simulink model "KINARM_Dyn_Inv"  (Simulink 8.7)
settings: Solver=ode45  StartTime=tSimStart  StopTime=tSimEnd  FixedStep=0.005  RelTol=1e-24  AbsTol=1e-24  SampleTimeConstraint=STIndependent
undefined symbols (not defined in the file or in its folder): g, IeR, IsR, iStep, IwR, me, ms, mw, nIC
libraries: mblibv1 x28
Description:
  | MSB - Demo 2
settings Model: Creator=arnav  LastModifiedBy=LAB  ExtModeAutoUpdateStatusClock=off
settings SolverCC: InitialStep=iStep  ShapePreserveControl=EnableAll  ZeroCrossControl=EnableAll  ZeroCrossAlgorithm=Adaptive
settings DataIOCC: ExternalInput=[smpltime]  SignalLoggingSaveFormat=ModelDataLogs  SaveOutput=off  SignalLogging=off  DSMLogging=off  SaveTime=off  SignalLoggingName=sigsOut  Refine=5
settings OptimizationCC: BooleanDataType=off  ExpressionDepthLimit=2147483647  InitFltsAndDblsToZero=on
settings DebuggingCC: SaveWithParameterizedLinksMsg=none  CheckExecutionContextPreStartOutputMsg=on  CheckExecutionContextRuntimeOutputMsg=on  SignalResolutionControl=TryResolveAllWithWarning  MultiTaskDSMMsg=warning  MultiTaskCondExecSysMsg=none  FcnCallInpInsideContextMsg=UseLocalSettings  UnconnectedInputMsg=none  UnconnectedOutputMsg=none  UnconnectedLineMsg=none  StateNameClashWarn=warning
settings HardwareCC: TargetUnknown=on
settings GRTTargetCC: TargetFcnLib=ansi_tfl_tmw.mat  CombineOutputUpdateFcns=off  GRTInterface=on
settings ConfigurationSet: Description=SimMechanics 2G

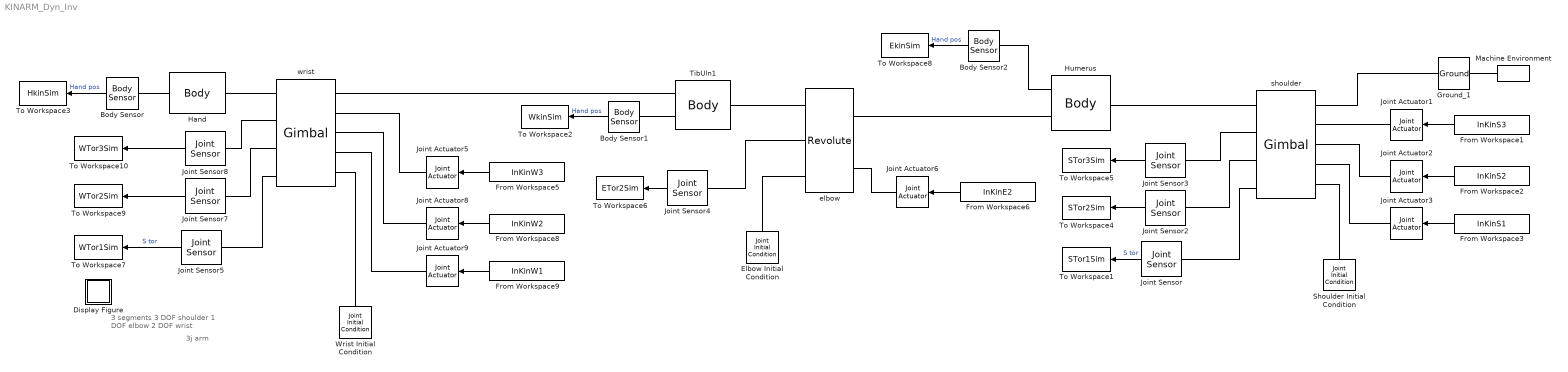
== system KINARM_Dyn_Inv ==
  note: 3j arm
  note: 3 segments
      | 3 DOF shoulder
      | 1 DOF elbow
      | 2 DOF wrist
  Body Sensor : mblibv1/Sensors &  Actuators/Body Sensor  UpdateFromCAD=off  PhysicalDomain=Mechanical  PortType=blob  Muxed=on  Pose=off  Angle=on  AngleUnits=deg  ArcVelocity=off  ArcVelocityUnits=deg/s  ArcAcceleration=off  ArcAccelerationUnits=deg/s^2  CoordPosition=on  CoordPositionUnits=m  Velocity=off  VelocityUnits=m/s  Acceleration=off  AccelerationUnits=m/s^2  Quaternion=on  QuaternionDT=off  QuaternionDDT=off  QuaternionUnits=off  OutputVector=[ 3 ]  ActiveIO=on  Width=3  DialogClass=MechanicalSensorBlock  ReferenceFrame=Absolute (World)
  Body Sensor1 : mblibv1/Sensors &  Actuators/Body Sensor  UpdateFromCAD=off  PhysicalDomain=Mechanical  PortType=blob  Muxed=on  Pose=off  Angle=on  AngleUnits=deg  ArcVelocity=off  ArcVelocityUnits=deg/s  ArcAcceleration=off  ArcAccelerationUnits=deg/s^2  CoordPosition=on  CoordPositionUnits=m  Velocity=off  VelocityUnits=m/s  Acceleration=off  AccelerationUnits=m/s^2  Quaternion=on  QuaternionDT=off  QuaternionDDT=off  QuaternionUnits=off  OutputVector=[ 3 ]  ActiveIO=on  Width=3  DialogClass=MechanicalSensorBlock  ReferenceFrame=Absolute (World)
  Body Sensor2 : mblibv1/Sensors &  Actuators/Body Sensor  UpdateFromCAD=off  PhysicalDomain=Mechanical  PortType=blob  Muxed=on  Pose=off  Angle=on  AngleUnits=deg  ArcVelocity=off  ArcVelocityUnits=deg/s  ArcAcceleration=off  ArcAccelerationUnits=deg/s^2  CoordPosition=on  CoordPositionUnits=m  Velocity=off  VelocityUnits=m/s  Acceleration=off  AccelerationUnits=m/s^2  Quaternion=on  QuaternionDT=off  QuaternionDDT=off  QuaternionUnits=off  OutputVector=[ 3 ]  ActiveIO=on  Width=3  DialogClass=MechanicalSensorBlock  ReferenceFrame=Absolute (World)
  Display Figure : Subsystem  Tag=Help  Description="Help callback for four bar model: mech_four_bar.  Opens Help browser to Type 19 marker at documentation for this tutorial model."  mask(Help callback){}
      settings: OpenFcn=pmhelpview([docroot '/toolbox/physmod/mech/mech.map'], 'mech_four_bar_help');
      mask Display: image(imread('info.bmp'))
  Elbow Initial Condition : mblibv1/Sensors &  Actuators/Joint Initial Condition  UpdateFromCAD=off  LeftPortType=blob  RightPortType=blob  PhysicalDomain=mechanical  DialogClass=InitialConditionBlock  InitialConditions=P1$false$0$m$deg$0$m/s$deg/s#P2$false$0$m$deg$0$m/s$deg/s#P3$false$0$m$deg$0$m/s$deg/s#R1$true$nIC(4,1)$m$rad$nIC(4,2)$m/s$rad/s#R2$false$nKin(1,1,5)$m$rad$nKin(1,2,5)$m/s$rad/s#R3$false$nKin(1,1,6)$m$rad$nKin(1,2,6)$m/s$rad/s#S$false$0$m$deg$0$m/s$deg/s  P1PIC=0  P1VIC=0  P2PIC=0  P2VIC=0  P3PIC=0  P3VIC=0  R1PIC=nIC(4,1)  R1VIC=nIC(4,2)  R2PIC=0  R2VIC=0  R3PIC=0  R3VIC=0  SPIC=0  SVIC=0
  From Workspace1 : FromWorkspace  VariableName=InKinS3  SampleTime=iStep  OutputAfterFinalValue=Holding final value
  From Workspace2 : FromWorkspace  VariableName=InKinS2  SampleTime=iStep  OutputAfterFinalValue=Holding final value
  From Workspace3 : FromWorkspace  VariableName=InKinS1  SampleTime=iStep  OutputAfterFinalValue=Holding final value
  From Workspace5 : FromWorkspace  VariableName=InKinW3  SampleTime=iStep  OutputAfterFinalValue=Holding final value
  From Workspace6 : FromWorkspace  VariableName=InKinE2  SampleTime=iStep  OutputAfterFinalValue=Holding final value
  From Workspace8 : FromWorkspace  VariableName=InKinW2  SampleTime=iStep  OutputAfterFinalValue=Holding final value
  From Workspace9 : FromWorkspace  VariableName=InKinW1  SampleTime=iStep  OutputAfterFinalValue=Holding final value
  Ground_1 : mblibv1/Bodies/Ground  UpdateFromCAD=off  LeftPortType=env  RightPortType=workingframe  PhysicalDomain=Mechanical  DialogClass=GroundBlock  CoordPosition=Spos  CoordPositionUnits=m  StateVectorMgrId=0  MachineId=[1 0]  ShowEnvPort=on  ParameterChecksum=[490472178, 4116704370, 4112686805, 3275683724]  TopologyChecksum=[4125622607, 929092055, 1872909337, 165519805]
  Hand : mblibv1/Bodies/Body  LConnTagsString=CS4  RConnTagsString=CS3  UpdateFromCAD=off  DialogClass=MechanicalBodyBlock  Mass=mw  MassUnits=kg  InertiaUnits=kg*m^2  Inertia=IwR  Shape=Cylinder  ShapeDims=[1 1]  ShapeUnits=m  ShapeUse=false  Density=1  DensityUnits=kg/m^3  DensityUse=false  GraphicsMode=MACHINE_DEFAULT  BodyColorSelMode=MACHINE_DEFAULT  BodyColor=[1 0 0]  AttachedToCS=CG  CG=Left$CG$HposCM$CS3$CS3$m$[0 0 0]$Euler X-Z-X$deg$WORLD$false$none  WorkingFrames=Right$CS3$Wpos$World$World$m$[0 0 0]$Euler X-Y-Z$deg$Adjoining$true$none#Left$CS4$Hpos$World$World$m$[0 0 0]$Euler X-Y-Z$deg$WORLD$true$none#Left$CS8$[0 0 0]$CS4$CS4$m$[0 0 0]$Euler X-Y-Z$deg$WORLD$false$none#Left$CS7$[0 0 0]$CS4$CS4$m$[0 0 0]$Euler X-Y-Z$deg$WORLD$false$none#Left$CS6$[0 0 0]$CS4$CS4$m$[0 0 0]$Euler X-Y-Z$deg$WORLD$false$none  CGPos=HposCM  CGRot=[0 0 0]  CS0Pos=[]  CS0Rot=[]  CS1Pos=[]  CS1Rot=[]  CS2Pos=[]  CS2Rot=[]  CS3Pos=Wpos  CS3Rot=[0 0 0]  CS4Pos=Hpos  CS4Rot=[0 0 0]  CS5Pos=[]  CS5Rot=[]  CS6Pos=[0 0 0]  CS6Rot=[0 0 0]  CS7Pos=[0 0 0]  CS7Rot=[0 0 0]  CS8Pos=[0 0 0]  CS8Rot=[0 0 0]  CS9Pos=[]  CS9Rot=[]  CS10Pos=[]  CS10Rot=[]  CS11Pos=[]  CS11Rot=[]  CS12Pos=[]  CS12Rot=[]  CS13Pos=[]  CS13Rot=[]  CS14Pos=[]  CS14Rot=[]  CS15Pos=[]  CS15Rot=[]  CS16Pos=[]  CS16Rot=[]  CS17Pos=[]  CS17Rot=[]  CS18Pos=[]  CS18Rot=[]  CS19Pos=[]  CS19Rot=[]  CS20Pos=[]  CS20Rot=[]
  Humerus : mblibv1/Bodies/Body  LConnTagsString=CS1  RConnTagsString=CS3|CS2  UpdateFromCAD=off  DialogClass=MechanicalBodyBlock  Mass=ms  MassUnits=kg  InertiaUnits=kg*m^2  Inertia=IsR  Shape=Cylinder  ShapeDims=[1 1]  ShapeUnits=m  ShapeUse=false  Density=1  DensityUnits=kg/m^3  DensityUse=false  GraphicsMode=MACHINE_DEFAULT  BodyColorSelMode=MACHINE_DEFAULT  BodyColor=[1 0 0]  AttachedToCS=CG  CG=Left$CG$EposCM$World$World$m$[0 0 0]$Euler X-Y-Z$deg$WORLD$false$none  WorkingFrames=Left$CS1$Spos$WORLD$WORLD$m$[0 0 0]$Euler X-Y-Z$deg$WORLD$true$none#Left$CS4$Spos$WORLD$WORLD$m$[0 0 0]$Euler X-Y-Z$deg$WORLD$false$none#Right$CS3$Epos$WORLD$WORLD$m$[0 0 0]$Euler X-Y-Z$deg$WORLD$true$none#Right$CS2$Epos$World$World$m$[0 0 0]$Euler X-Y-Z$deg$WORLD$true$none  CGPos=EposCM  CGRot=[0 0 0]  CS0Pos=[]  CS0Rot=[]  CS1Pos=Spos  CS1Rot=[0 0 0]  CS2Pos=Epos  CS2Rot=[0 0 0]  CS3Pos=Epos  CS3Rot=[0 0 0]  CS4Pos=Spos  CS4Rot=[0 0 0]  CS5Pos=[]  CS5Rot=[]  CS6Pos=[]  CS6Rot=[]  CS7Pos=[]  CS7Rot=[]  CS8Pos=[]  CS8Rot=[]  CS9Pos=[]  CS9Rot=[]  CS10Pos=[]  CS10Rot=[]  CS11Pos=[]  CS11Rot=[]  CS12Pos=[]  CS12Rot=[]  CS13Pos=[]  CS13Rot=[]  CS14Pos=[]  CS14Rot=[]  CS15Pos=[]  CS15Rot=[]  CS16Pos=[]  CS16Rot=[]  CS17Pos=[]  CS17Rot=[]  CS18Pos=[]  CS18Rot=[]  CS19Pos=[]  CS19Rot=[]  CS20Pos=[]  CS20Rot=[]
  Joint Actuator1 : mblibv1/Sensors &  Actuators/Joint Actuator  UpdateFromCAD=off  PhysicalDomain=Mechanical  PortType=blob  ActuationStyle=Motion  AngleUnits=rad  ArcVelocityUnits=rad/s  ArcAccelerationUnits=rad/s^2  CoordPositionUnits=m  VelocityUnits=m/s  AccelerationUnits=m/s^2  ForceUnits=N  TorqueUnits=N*m  ActiveIO=on  Width=3  DialogClass=MechanicalActuatorBlock  Primitive=R3  ReferenceFrame=Absolute (INERTIAL)
  Joint Actuator2 : mblibv1/Sensors &  Actuators/Joint Actuator  UpdateFromCAD=off  PhysicalDomain=Mechanical  PortType=blob  ActuationStyle=Motion  AngleUnits=rad  ArcVelocityUnits=rad/s  ArcAccelerationUnits=rad/s^2  CoordPositionUnits=m  VelocityUnits=m/s  AccelerationUnits=m/s^2  ForceUnits=N  TorqueUnits=N*m  ActiveIO=on  Width=3  DialogClass=MechanicalActuatorBlock  Primitive=R2  ReferenceFrame=Absolute (INERTIAL)
  Joint Actuator3 : mblibv1/Sensors &  Actuators/Joint Actuator  UpdateFromCAD=off  PhysicalDomain=Mechanical  PortType=blob  ActuationStyle=Motion  AngleUnits=rad  ArcVelocityUnits=rad/s  ArcAccelerationUnits=rad/s^2  CoordPositionUnits=m  VelocityUnits=m/s  AccelerationUnits=m/s^2  ForceUnits=N  TorqueUnits=N*m  ActiveIO=on  Width=3  DialogClass=MechanicalActuatorBlock  Primitive=R1  ReferenceFrame=Absolute (INERTIAL)
  Joint Actuator5 : mblibv1/Sensors &  Actuators/Joint Actuator  UpdateFromCAD=off  PhysicalDomain=Mechanical  PortType=blob  ActuationStyle=Motion  AngleUnits=rad  ArcVelocityUnits=rad/s  ArcAccelerationUnits=rad/s^2  CoordPositionUnits=m  VelocityUnits=m/s  AccelerationUnits=m/s^2  ForceUnits=N  TorqueUnits=N*m  ActiveIO=on  Width=3  DialogClass=MechanicalActuatorBlock  Primitive=R3  ReferenceFrame=Absolute (INERTIAL)
  Joint Actuator6 : mblibv1/Sensors &  Actuators/Joint Actuator  UpdateFromCAD=off  PhysicalDomain=Mechanical  PortType=blob  ActuationStyle=Motion  AngleUnits=rad  ArcVelocityUnits=rad/s  ArcAccelerationUnits=rad/s^2  CoordPositionUnits=m  VelocityUnits=m/s  AccelerationUnits=m/s^2  ForceUnits=N  TorqueUnits=N*m  ActiveIO=on  Width=3  DialogClass=MechanicalActuatorBlock  Primitive=R1  ReferenceFrame=Absolute (INERTIAL)
  Joint Actuator8 : mblibv1/Sensors &  Actuators/Joint Actuator  UpdateFromCAD=off  PhysicalDomain=Mechanical  PortType=blob  ActuationStyle=Motion  AngleUnits=rad  ArcVelocityUnits=rad/s  ArcAccelerationUnits=rad/s^2  CoordPositionUnits=m  VelocityUnits=m/s  AccelerationUnits=m/s^2  ForceUnits=N  TorqueUnits=N*m  ActiveIO=on  Width=3  DialogClass=MechanicalActuatorBlock  Primitive=R2  ReferenceFrame=Absolute (INERTIAL)
  Joint Actuator9 : mblibv1/Sensors &  Actuators/Joint Actuator  UpdateFromCAD=off  PhysicalDomain=Mechanical  PortType=blob  ActuationStyle=Motion  AngleUnits=rad  ArcVelocityUnits=rad/s  ArcAccelerationUnits=rad/s^2  CoordPositionUnits=m  VelocityUnits=m/s  AccelerationUnits=m/s^2  ForceUnits=N  TorqueUnits=N*m  ActiveIO=on  Width=3  DialogClass=MechanicalActuatorBlock  Primitive=R1  ReferenceFrame=Absolute (INERTIAL)
  Joint Sensor : mblibv1/Sensors &  Actuators/Joint Sensor  UpdateFromCAD=off  PhysicalDomain=Mechanical  PortType=blob  Muxed=off  Pose=off  Angle=off  AngleUnits=rad  ArcVelocity=off  ArcVelocityUnits=rad/s  ArcAcceleration=off  ArcAccelerationUnits=rad/s^2  CoordPosition=on  CoordPositionUnits=m  Velocity=off  VelocityUnits=m/s  Acceleration=off  AccelerationUnits=m/s^2  Quaternion=on  QuaternionDT=off  QuaternionDDT=off  QuaternionUnits=off  OutputVector=[ 1 1 ]  ActiveIO=on  Width=1  DialogClass=MechanicalSensorBlock  Primitive=R1  Force=off  ForceUnits=N  Torque=on  TorqueUnits=N*m  ReferenceFrame=Absolute (INERTIAL)  ReactionSensedSide=Base  ReactionReferenceFrame=Local (Body CS)  ReactionForce=off  ReactionForceUnits=N  ReactionMoment=off  ReactionMomentUnits=N*m
  Joint Sensor2 : mblibv1/Sensors &  Actuators/Joint Sensor  UpdateFromCAD=off  PhysicalDomain=Mechanical  PortType=blob  Muxed=off  Pose=off  Angle=off  AngleUnits=rad  ArcVelocity=off  ArcVelocityUnits=rad/s  ArcAcceleration=off  ArcAccelerationUnits=rad/s^2  CoordPosition=on  CoordPositionUnits=m  Velocity=off  VelocityUnits=m/s  Acceleration=off  AccelerationUnits=m/s^2  Quaternion=on  QuaternionDT=off  QuaternionDDT=off  QuaternionUnits=off  OutputVector=[ 1 1 ]  ActiveIO=on  Width=1  DialogClass=MechanicalSensorBlock  Primitive=R2  Force=off  ForceUnits=N  Torque=on  TorqueUnits=N*m  ReferenceFrame=Absolute (INERTIAL)  ReactionSensedSide=Base  ReactionReferenceFrame=Local (Body CS)  ReactionForce=off  ReactionForceUnits=N  ReactionMoment=off  ReactionMomentUnits=N*m
  Joint Sensor3 : mblibv1/Sensors &  Actuators/Joint Sensor  UpdateFromCAD=off  PhysicalDomain=Mechanical  PortType=blob  Muxed=off  Pose=off  Angle=off  AngleUnits=rad  ArcVelocity=off  ArcVelocityUnits=rad/s  ArcAcceleration=off  ArcAccelerationUnits=rad/s^2  CoordPosition=on  CoordPositionUnits=m  Velocity=off  VelocityUnits=m/s  Acceleration=off  AccelerationUnits=m/s^2  Quaternion=on  QuaternionDT=off  QuaternionDDT=off  QuaternionUnits=off  OutputVector=[ 1 1 ]  ActiveIO=on  Width=1  DialogClass=MechanicalSensorBlock  Primitive=R3  Force=off  ForceUnits=N  Torque=on  TorqueUnits=N*m  ReferenceFrame=Absolute (INERTIAL)  ReactionSensedSide=Base  ReactionReferenceFrame=Local (Body CS)  ReactionForce=off  ReactionForceUnits=N  ReactionMoment=off  ReactionMomentUnits=N*m
  Joint Sensor4 : mblibv1/Sensors &  Actuators/Joint Sensor  UpdateFromCAD=off  PhysicalDomain=Mechanical  PortType=blob  Muxed=off  Pose=off  Angle=off  AngleUnits=rad  ArcVelocity=off  ArcVelocityUnits=rad/s  ArcAcceleration=off  ArcAccelerationUnits=rad/s^2  CoordPosition=on  CoordPositionUnits=m  Velocity=off  VelocityUnits=m/s  Acceleration=off  AccelerationUnits=m/s^2  Quaternion=on  QuaternionDT=off  QuaternionDDT=off  QuaternionUnits=off  OutputVector=[ 1 1 ]  ActiveIO=on  Width=1  DialogClass=MechanicalSensorBlock  Primitive=R1  Force=off  ForceUnits=N  Torque=on  TorqueUnits=N*m  ReferenceFrame=Absolute (INERTIAL)  ReactionSensedSide=Base  ReactionReferenceFrame=Local (Body CS)  ReactionForce=off  ReactionForceUnits=N  ReactionMoment=off  ReactionMomentUnits=N*m
  Joint Sensor5 : mblibv1/Sensors &  Actuators/Joint Sensor  UpdateFromCAD=off  PhysicalDomain=Mechanical  PortType=blob  Muxed=off  Pose=off  Angle=off  AngleUnits=rad  ArcVelocity=off  ArcVelocityUnits=rad/s  ArcAcceleration=off  ArcAccelerationUnits=rad/s^2  CoordPosition=on  CoordPositionUnits=m  Velocity=off  VelocityUnits=m/s  Acceleration=off  AccelerationUnits=m/s^2  Quaternion=on  QuaternionDT=off  QuaternionDDT=off  QuaternionUnits=off  OutputVector=[ 1 1 ]  ActiveIO=on  Width=1  DialogClass=MechanicalSensorBlock  Primitive=R1  Force=off  ForceUnits=N  Torque=on  TorqueUnits=N*m  ReferenceFrame=Absolute (INERTIAL)  ReactionSensedSide=Base  ReactionReferenceFrame=Local (Body CS)  ReactionForce=off  ReactionForceUnits=N  ReactionMoment=off  ReactionMomentUnits=N*m
  Joint Sensor7 : mblibv1/Sensors &  Actuators/Joint Sensor  UpdateFromCAD=off  PhysicalDomain=Mechanical  PortType=blob  Muxed=off  Pose=off  Angle=off  AngleUnits=rad  ArcVelocity=off  ArcVelocityUnits=rad/s  ArcAcceleration=off  ArcAccelerationUnits=rad/s^2  CoordPosition=on  CoordPositionUnits=m  Velocity=off  VelocityUnits=m/s  Acceleration=off  AccelerationUnits=m/s^2  Quaternion=on  QuaternionDT=off  QuaternionDDT=off  QuaternionUnits=off  OutputVector=[ 1 1 ]  ActiveIO=on  Width=1  DialogClass=MechanicalSensorBlock  Primitive=R2  Force=off  ForceUnits=N  Torque=on  TorqueUnits=N*m  ReferenceFrame=Absolute (INERTIAL)  ReactionSensedSide=Base  ReactionReferenceFrame=Local (Body CS)  ReactionForce=off  ReactionForceUnits=N  ReactionMoment=off  ReactionMomentUnits=N*m
  Joint Sensor8 : mblibv1/Sensors &  Actuators/Joint Sensor  UpdateFromCAD=off  PhysicalDomain=Mechanical  PortType=blob  Muxed=off  Pose=off  Angle=off  AngleUnits=rad  ArcVelocity=off  ArcVelocityUnits=rad/s  ArcAcceleration=off  ArcAccelerationUnits=rad/s^2  CoordPosition=on  CoordPositionUnits=m  Velocity=off  VelocityUnits=m/s  Acceleration=off  AccelerationUnits=m/s^2  Quaternion=on  QuaternionDT=off  QuaternionDDT=off  QuaternionUnits=off  OutputVector=[ 1 1 ]  ActiveIO=on  Width=1  DialogClass=MechanicalSensorBlock  Primitive=R3  Force=off  ForceUnits=N  Torque=on  TorqueUnits=N*m  ReferenceFrame=Absolute (INERTIAL)  ReactionSensedSide=Base  ReactionReferenceFrame=Local (Body CS)  ReactionForce=off  ReactionForceUnits=N  ReactionMoment=off  ReactionMomentUnits=N*m
  Machine Environment : mblibv1/Bodies/Machine Environment  Tag=Factory ground  PortType=env  PhysicalDomain=Mechanical  DialogTemplateClass=MECH.MachineEnvironment  SyncWhenCopied=off  Gravity=[0 0 -g]  GravityUnits=m/s^2  GravityAsSignal=off  Dimensionality=3D Only  AnalysisType=Inverse dynamics  LinearAssemblyTolerance=1e-12  LinearAssemblyToleranceUnits=m  AngularAssemblyTolerance=1e-12  AngularAssemblyToleranceUnits=rad  ConstraintSolverType=Stabilizing  ConstraintRelTolerance=1e-4  ConstraintAbsTolerance=1e-4  UseRobustSingularityHandling=off  RedundancyAnalysisToleranceType=Automatically select tolerance  RedundancyAnalysisTolerance=1e-14  StatePerturbationType=Adaptive  PerturbationSize=1e-3  VisualizeMachine=off  BodyVisualizationType=Convex hull from body CS locations  BodyColorSelMode=Use model default  DefaultBodyColor=[1 0 0]
  Shoulder Initial Condition : mblibv1/Sensors &  Actuators/Joint Initial Condition  UpdateFromCAD=off  LeftPortType=blob  RightPortType=blob  PhysicalDomain=mechanical  DialogClass=InitialConditionBlock  InitialConditions=P1$false$0$m$deg$0$m/s$deg/s#P2$false$0$m$deg$0$m/s$deg/s#P3$false$0$m$deg$0$m/s$deg/s#R1$true$nIC(1,1)$m$rad$nIC(1,2)$m/s$rad/s#R2$true$nIC(2,1)$m$rad$nIC(2,2)$m/s$rad/s#R3$true$nIC(3,1)$m$rad$nIC(3,2)$m/s$rad/s#S$false$0$m$deg$0$m/s$deg/s  P1PIC=0  P1VIC=0  P2PIC=0  P2VIC=0  P3PIC=0  P3VIC=0  R1PIC=nIC(1,1)  R1VIC=nIC(1,2)  R2PIC=nIC(2,1)  R2VIC=nIC(2,2)  R3PIC=nIC(3,1)  R3VIC=nIC(3,2)  SPIC=0  SVIC=0
  TibUln1 : mblibv1/Bodies/Body  LConnTagsString=CS3  RConnTagsString=CS4|CS5  UpdateFromCAD=off  DialogClass=MechanicalBodyBlock  Mass=me  MassUnits=kg  InertiaUnits=kg*m^2  Inertia=IeR  Shape=Cylinder  ShapeDims=[1 1]  ShapeUnits=m  ShapeUse=false  Density=1  DensityUnits=kg/m^3  DensityUse=false  GraphicsMode=MACHINE_DEFAULT  BodyColorSelMode=MACHINE_DEFAULT  BodyColor=[1 0 0]  AttachedToCS=CG  CG=Left$CG$WposCM$CS3$CS3$m$[0 0 0]$Euler X-Z-X$deg$WORLD$false$none  WorkingFrames=Left$CS3$Epos$World$World$m$[0 0 0]$Euler X-Y-Z$deg$Adjoining$true$none#Right$CS4$Wpos$World$World$m$[0 0 0]$Euler X-Y-Z$deg$WORLD$true$none#Right$CS5$Wpos$World$World$m$[0 0 0]$Euler X-Y-Z$deg$WORLD$true$none  CGPos=WposCM  CGRot=[0 0 0]  CS0Pos=[]  CS0Rot=[]  CS1Pos=[]  CS1Rot=[]  CS2Pos=[]  CS2Rot=[]  CS3Pos=Epos  CS3Rot=[0 0 0]  CS4Pos=Wpos  CS4Rot=[0 0 0]  CS5Pos=Wpos  CS5Rot=[0 0 0]  CS6Pos=[]  CS6Rot=[]  CS7Pos=[]  CS7Rot=[]  CS8Pos=[]  CS8Rot=[]  CS9Pos=[]  CS9Rot=[]  CS10Pos=[]  CS10Rot=[]  CS11Pos=[]  CS11Rot=[]  CS12Pos=[]  CS12Rot=[]  CS13Pos=[]  CS13Rot=[]  CS14Pos=[]  CS14Rot=[]  CS15Pos=[]  CS15Rot=[]  CS16Pos=[]  CS16Rot=[]  CS17Pos=[]  CS17Rot=[]  CS18Pos=[]  CS18Rot=[]  CS19Pos=[]  CS19Rot=[]  CS20Pos=[]  CS20Rot=[]
  To Workspace1 : ToWorkspace  VariableName=STor1Sim  SaveFormat=Structure With Time  SampleTime=-1
      settings: Decimation=5
  To Workspace10 : ToWorkspace  VariableName=WTor3Sim  SaveFormat=Structure With Time  SampleTime=-1
      settings: Decimation=5
  To Workspace2 : ToWorkspace  VariableName=WkinSim  SampleTime=-1
      settings: Decimation=5
  To Workspace3 : ToWorkspace  VariableName=HkinSim  SampleTime=-1
      settings: Decimation=5
  To Workspace4 : ToWorkspace  VariableName=STor2Sim  SaveFormat=Structure With Time  SampleTime=-1
      settings: Decimation=5
  To Workspace5 : ToWorkspace  VariableName=STor3Sim  SaveFormat=Structure With Time  SampleTime=-1
      settings: Decimation=5
  To Workspace6 : ToWorkspace  VariableName=ETor2Sim  SaveFormat=Structure With Time  SampleTime=-1
      settings: Decimation=5
  To Workspace7 : ToWorkspace  VariableName=WTor1Sim  SaveFormat=Structure With Time  SampleTime=-1
      settings: Decimation=5
  To Workspace8 : ToWorkspace  VariableName=EkinSim  SampleTime=-1
      settings: Decimation=5
  To Workspace9 : ToWorkspace  VariableName=WTor2Sim  SaveFormat=Structure With Time  SampleTime=-1
      settings: Decimation=5
  Wrist Initial Condition : mblibv1/Sensors &  Actuators/Joint Initial Condition  UpdateFromCAD=off  LeftPortType=blob  RightPortType=blob  PhysicalDomain=mechanical  DialogClass=InitialConditionBlock  InitialConditions=P1$false$0$m$deg$0$m/s$deg/s#P2$false$0$m$deg$0$m/s$deg/s#P3$false$0$m$deg$0$m/s$deg/s#R1$true$nIC(5,1)$m$rad$nIC(5,2)$m/s$rad/s#R2$true$nIC(6,1)$m$rad$nIC(6,2)$m/s$rad/s#R3$true$nIC(7,1)$m$rad$nIC(7,2)$m/s$rad/s#S$false$0$m$deg$0$m/s$deg/s  P1PIC=0  P1VIC=0  P2PIC=0  P2VIC=0  P3PIC=0  P3VIC=0  R1PIC=nIC(5,1)  R1VIC=nIC(5,2)  R2PIC=nIC(6,1)  R2VIC=nIC(6,2)  R3PIC=nIC(7,1)  R3VIC=nIC(7,2)  SPIC=0  SVIC=0
  elbow : mblibv1/Joints/Revolute  LConnTagsString=__newl0|SA1|SA2  RConnTagsString=__newr0|SA1  UpdateFromCAD=off  NumSAPorts=3  CutJoint=off  MarkAsCut=off  Primitives=prismatic  PrimitiveProps=R1$Base$[1 0 0]$revolute  DialogClass=JointBlock  R1Axis=[1 0 0]
  shoulder : mblibv1/Joints/Gimbal  LConnTagsString=__newl0|SA1|SA2|SA3|SA4  RConnTagsString=__newr0|SA1|SA2|SA3  UpdateFromCAD=off  NumSAPorts=7  CutJoint=off  MarkAsCut=off  Primitives=prismatic_prismatic  PrimitiveProps=R1$Base$[1 0 0]$revolute#R2$Base$[0 1 0]$revolute#R3$Base$[0 0 1]$revolute  DialogClass=JointBlock  R1Axis=[1 0 0]  R2Axis=[0 1 0]  R3Axis=[0 0 1]
  wrist : mblibv1/Joints/Gimbal  LConnTagsString=__newl0|SA1|SA2|SA3|SA4  RConnTagsString=__newr0|SA1|SA2|SA3  UpdateFromCAD=off  NumSAPorts=7  CutJoint=off  MarkAsCut=off  Primitives=prismatic_prismatic  PrimitiveProps=R1$Base$[1 0 0]$revolute#R2$Base$[0 1 0]$revolute#R3$Base$[0 0 1]$revolute  DialogClass=JointBlock  R1Axis=[1 0 0]  R2Axis=[0 1 0]  R3Axis=[0 0 1]
  wires:
  Body Sensor/1 -> To Workspace3/1  "Hand pos"
  From Workspace1/1 -> Joint Actuator1/1
  Joint Sensor/1 -> To Workspace1/1  "S tor"
  From Workspace2/1 -> Joint Actuator2/1
  Joint Sensor2/1 -> To Workspace4/1
  From Workspace3/1 -> Joint Actuator3/1
  Joint Sensor3/1 -> To Workspace5/1
  From Workspace6/1 -> Joint Actuator6/1
  Joint Sensor4/1 -> To Workspace6/1
  From Workspace5/1 -> Joint Actuator5/1
  Joint Sensor5/1 -> To Workspace7/1  "S tor"
  From Workspace8/1 -> Joint Actuator8/1
  Joint Sensor7/1 -> To Workspace9/1
  From Workspace9/1 -> Joint Actuator9/1
  Joint Sensor8/1 -> To Workspace10/1
  Body Sensor1/1 -> To Workspace2/1  "Hand pos"
  Body Sensor2/1 -> To Workspace8/1  "Hand pos"
  connections:
  Machine Environment/RConn1 -- Ground_1/LConn1
  Ground_1/RConn1 -- shoulder/LConn1
  Joint Sensor/LConn1 -- shoulder/RConn4
  Joint Sensor2/LConn1 -- shoulder/RConn3
  Joint Sensor3/LConn1 -- shoulder/RConn2
  Joint Actuator1/RConn1 -- shoulder/LConn2
  Joint Actuator2/RConn1 -- shoulder/LConn3
  Joint Actuator3/RConn1 -- shoulder/LConn4
  Shoulder Initial Condition/RConn1 -- shoulder/LConn5
  elbow/RConn2 -- Joint Actuator6/RConn1
  elbow/RConn1 -- Humerus/RConn2
  shoulder/RConn1 -- Humerus/LConn1
  Joint Actuator5/RConn1 -- wrist/LConn2
  Wrist Initial Condition/RConn1 -- wrist/LConn5
  Joint Actuator8/RConn1 -- wrist/LConn3
  Joint Actuator9/RConn1 -- wrist/LConn4
  Joint Sensor5/LConn1 -- wrist/RConn4
  Joint Sensor7/LConn1 -- wrist/RConn3
  Joint Sensor8/LConn1 -- wrist/RConn2
  elbow/LConn1 -- TibUln1/LConn1
  TibUln1/RConn1 -- wrist/LConn1
  Body Sensor/LConn1 -- Hand/LConn1
  Hand/RConn1 -- wrist/RConn1
  Joint Sensor4/LConn1 -- elbow/LConn2
  Elbow Initial Condition/RConn1 -- elbow/LConn3
  Body Sensor1/LConn1 -- TibUln1/RConn2
  Body Sensor2/LConn1 -- Humerus/RConn1

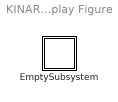
== system KINARM_Dyn_Inv/Display Figure ==
  EmptySubsystem : Subsystem

== system KINARM_Dyn_Inv/Display Figure/EmptySubsystem ==
